simulink model "muscleLegs_task1"  (R2025b)
settings: Solver=ode23t  StartTime=0.0  StopTime=t_end  MaxStep=1e-3  RelTol=1e-4
values from neighbouring files (symbols this model uses):
  c = 0.05    [setup_muscleLegs_nm.m]
  CtrlPar = [tau_H_st; phi_K_tgt_st; P_K_st; D_K_st ... (first row only)    [setup_muscleLegs_ctrl.m]
  eref_se = 0.04    [setup_muscleLegs_nm.m]
  FmaxBFSH = 350    [setup_muscleLegs_nm.m]
  FmaxGLU = 4000    [setup_muscleLegs_nm.m]
  FmaxHFL = 2000    [setup_muscleLegs_nm.m]
  FmaxVAS = 5000    [setup_muscleLegs_nm.m]
  g = 9.81    [setup_muscleLegs_model.m]
  init_stim = 0.01    [setup_muscleLegs_nm.m]
  K = 5    [setup_muscleLegs_nm.m]
  l_shank = l_leg/2    (= 0.49)    [setup_muscleLegs_model.m]
  l_thigh = l_leg/2    (= 0.49)    [setup_muscleLegs_model.m]
  loptBFSH = 0.12    [setup_muscleLegs_nm.m]
  loptGLU = 0.11    [setup_muscleLegs_nm.m]
  loptHFL = 0.11    [setup_muscleLegs_nm.m]
  loptVAS = 0.08    [setup_muscleLegs_nm.m]
  lslackBFSH = 0.10    (= 0.1)    [setup_muscleLegs_nm.m]
  lslackGLU = 0.13    [setup_muscleLegs_nm.m]
  lslackHFL = 0.10    (= 0.1)    [setup_muscleLegs_nm.m]
  lslackVAS = 0.23    [setup_muscleLegs_nm.m]
  m_body = m_total - 2*m_foot    (= 78)    [setup_muscleLegs_model.m]
  m_shank = 4    [setup_muscleLegs_model.m]
  m_thigh = 8    [setup_muscleLegs_model.m]
  N = 12    [cmaes_task1_2_set1.mat]    (also in cmaes_task1_2_set2.mat; cmaes_task2_2_set1.mat = 17; cmaes_task2_2_set2.mat = 17; cmaes_task3_crouch.mat = 17)
  phirefBFSH = 160*pi/180    (= 2.79252680319)    [setup_muscleLegs_nm.m]
  phirefGLU = 60*pi/180    (= 1.0471975512)    [setup_muscleLegs_nm.m]
  phirefHFL = 20*pi/180    (= 0.349065850399)    [setup_muscleLegs_nm.m]
  phirefVAS = 60*pi/180    (= 1.0471975512)    [setup_muscleLegs_nm.m]
  plane_height = 0.1    [setup_muscleLegs_model.m]
  plane_x = 100    [setup_muscleLegs_model.m]
  plane_z = 1    [setup_muscleLegs_model.m]
  r_foot = 0.01    [setup_muscleLegs_model.m]
  rBFSH = 0.04    [setup_muscleLegs_nm.m]
  rGLU = 0.08    [setup_muscleLegs_nm.m]
  rHFL = 0.08    [setup_muscleLegs_nm.m]
  rhoBFSH = 0.7    [setup_muscleLegs_nm.m]
  rhoGLU = 0.5    [setup_muscleLegs_nm.m]
  rhoHFL = 0.5    [setup_muscleLegs_nm.m]
  rhoVAS = 0.6    [setup_muscleLegs_nm.m]
  rVAS = 0.05    [setup_muscleLegs_nm.m]
  tau_act = 0.01    [setup_muscleLegs_nm.m]
  tau_deact = 0.04    [setup_muscleLegs_nm.m]
  vi_Ctrl_st = 1:4    [setup_muscleLegs_ctrl.m]
  vi_Ctrl_sw = 5:12    [setup_muscleLegs_ctrl.m]
  vmaxBFSH = 12    [setup_muscleLegs_nm.m]
  vmaxGLU = 12    [setup_muscleLegs_nm.m]
  vmaxHFL = 12    [setup_muscleLegs_nm.m]
  vmaxVAS = 12    [setup_muscleLegs_nm.m]
  w = 0.56    [setup_muscleLegs_nm.m]
  w_pe = w    (= 0.56)    [setup_muscleLegs_nm.m]
undefined symbols (not defined in the file or in its folder): l1, X, Y, Z
libraries: sm_lib x30, nesl_utility x17, simulink x1
(part 1 of 4)
settings Model: Creator=ssm04  LastModifiedBy=mayan
settings SolverCC: AlgebraicLoopSolver=TrustRegion
settings OptimizationCC: ReuseModelBlockBuffer=off
settings RTWCC: GPUComputeCapability=3.5
settings ExplorerConfigSet: InternalSimMechanicsExplorerSettings="<ExplorerConfiguration><canonicalview>planar_xy</canonicalview><AnimationSetting><BasePlaybackSpeed>1.0</BasePlaybackSpeed><PlaybackSpeedFactor>1.0</PlaybackSpeedFactor></AnimationSetting><TilePanel><TileInfo><Tiles Columns=\"1\" Count=\"1\" Rows=\"1\"><Column Weight=\"1\"/><Row Weight=\"1\"/><Tile Height=\"1\" Width=\"1\" X=\"0\" Y=\"0\"/></Tiles></TileInfo><SceneInfo><SceneViewer><BGColor><R>0.60000002384185791</R><G>0.60000002384185791</G><B>0.60000002384185791</B></BGColor><Camera><DoPerspective>off</DoPerspective><Position><X>5.32836294698793811</X><Y>0.88627330653474079</Y><Z>5.31412817539694871</Z></Position><Center><X>5.32836294698793811</X><Y>0.88627330653474079</Y><Z>2.38238317962213841e-09</Z></Center><Up><X>0</X><Y>1</Y><Z>0</Z></Up><ViewLimDist>1</ViewLimDist><YLim>2.08582257526475079</YLim><XLim>5.52596682264529182</XLim></Camera></SceneViewer></SceneInfo></TilePanel><MechEditorPanel><Cameras/><GfxPanelCameraMap/><VideoCreator><PlaybackSpeedRatio>1.0</PlaybackSpeedRatio><FrameRate>30</FrameRate><VideoFormat>Motion JPEG AVI</VideoFormat><FrameSize>auto</FrameSize></VideoCreator></MechEditorPanel></ExplorerConfiguration>"

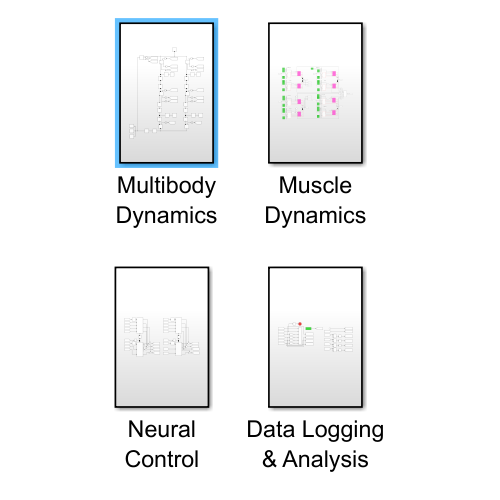
[thumbnail: Simulink's stored preview of the top-level diagram]
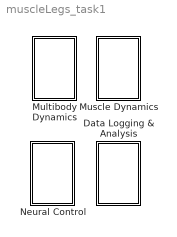
== system muscleLegs_task1 ==
  Data Logging & Analysis : Subsystem
  Multibody Dynamics : Subsystem
  Muscle Dynamics : Subsystem
  Neural Control : Subsystem

== system muscleLegs_task1/Data Logging & Analysis ==
  Clock : Clock
  Compare To Constant : simulink/Logic and Bit Operations/Compare To Constant  relop=<=  const=0.5  OutDataTypeStr=boolean
  Constant3 : Constant  Value=CtrlPar
  Divide{1..4} (4 alike) : Product
  Gain{,1..3} (4 alike) : Gain  Gain=180/pi
  Integrator{,1..3} (4 alike) : Integrator
  Scope1 : Scope  NumInputPorts=6
      settings: ActiveDisplayYMinimum=0.94241  ActiveDisplayYMaximum=1.51828
  Stop Simulation : Stop
  To Workspace : ToWorkspace  VariableName=t_end_sim  SaveFormat=Timeseries  SampleTime=-1
      settings: MaxDataPoints=1
  To Workspace1 : ToWorkspace  VariableName=x_end  SaveFormat=Timeseries  SampleTime=-1
      settings: MaxDataPoints=1
  To Workspace2 : ToWorkspace  VariableName=int_tau_H_L_2  SaveFormat=Timeseries  SampleTime=-1
      settings: MaxDataPoints=1
  To Workspace3 : ToWorkspace  VariableName=int_tau_K_L_2  SaveFormat=Timeseries  SampleTime=-1
      settings: MaxDataPoints=1
  To Workspace4 : ToWorkspace  VariableName=int_tau_H_R_2  SaveFormat=Timeseries  SampleTime=-1
      settings: MaxDataPoints=1
  To Workspace5 : ToWorkspace  VariableName=int_tau_K_R_2  SaveFormat=Timeseries  SampleTime=-1
      settings: MaxDataPoints=1
  To Workspace6 : ToWorkspace  VariableName=log_phi_H_L  SaveFormat=Timeseries  SampleTime=-1
  To Workspace7 : ToWorkspace  VariableName=log_phi_H_R  SaveFormat=Timeseries  SampleTime=-1
  To Workspace8 : ToWorkspace  VariableName=log_phi_K_L  SaveFormat=Timeseries  SampleTime=-1
  To Workspace9 : ToWorkspace  VariableName=log_phi_K_R  SaveFormat=Timeseries  SampleTime=-1
  tag scope: CtrlPar=global
  wires:
  Gain3/1 -> Scope1/6  "k_R"
  [body_y] -> Compare To Constant/1, Scope1/2
  [phi_K_L] -> To Workspace8/1, Gain1/1
  [tau_K_R] -> Divide3/2, Divide3/1
  Compare To Constant/1 -> Stop Simulation/1
  [phi_H_L] -> To Workspace6/1, Gain/1
  Integrator1/1 -> To Workspace3/1
  [phi_K_R] -> To Workspace9/1, Gain3/1
  [body_x] -> Scope1/1
  [tau_H_L] -> Divide2/2, Divide2/1
  Gain2/1 -> Scope1/5  "h_R"
  Gain/1 -> Scope1/3  "h_L"
  [phi_H_R] -> To Workspace7/1, Gain2/1
  [body_x] -> To Workspace1/1
  Clock/1 -> To Workspace/1
  Constant3/1 -> [CtrlPar]
  [tau_K_L] -> Divide1/2, Divide1/1
  Divide2/1 -> Integrator/1
  [tau_H_R] -> Divide4/2, Divide4/1
  Divide1/1 -> Integrator1/1
  Integrator3/1 -> To Workspace5/1
  Integrator2/1 -> To Workspace4/1
  Gain1/1 -> Scope1/4  "k_L"
  Divide4/1 -> Integrator2/1
  Integrator/1 -> To Workspace2/1
  Divide3/1 -> Integrator3/1

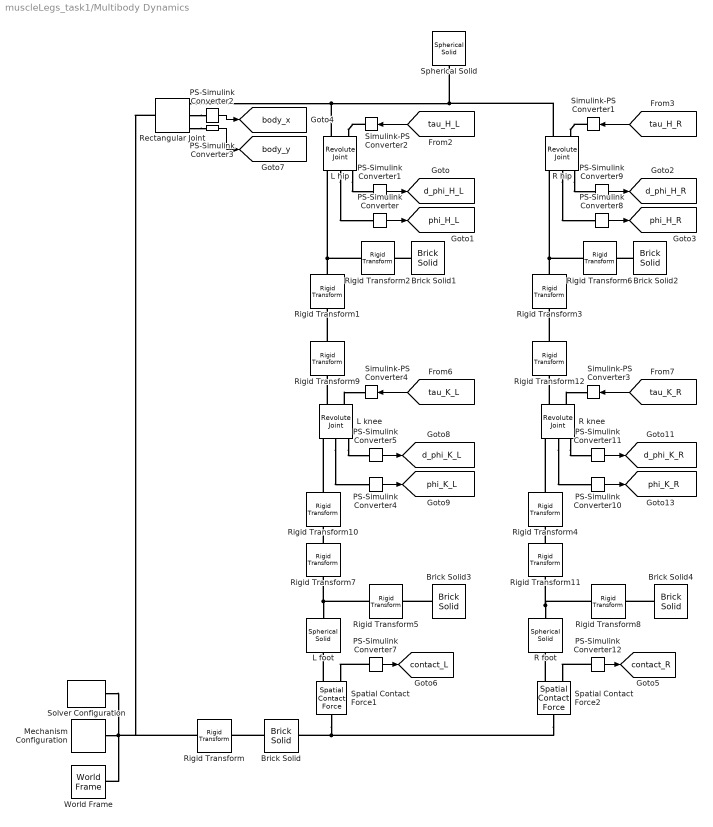
== system muscleLegs_task1/Multibody Dynamics ==
  Brick Solid : sm_lib/Body Elements/Brick Solid  BrickDimensions=[plane_x plane_height plane_z]  BrickDimensionsUnits=m  ExportEntireGeometry=on  InertiaType=CalculateFromGeometry  BasedOnType=Density  Density=1000  DensityUnits=kg/m^3  Mass=1  MassUnits=kg  CenterOfMass=[0 0 0]  CenterOfMassUnits=m  MomentsOfInertia=[1 1 1]  MomentsOfInertiaUnits=kg*m^2  ProductsOfInertia=[0 0 0]  ProductsOfInertiaUnits=kg*m^2  GraphicType=FromGeometry  MarkerShape=Sphere  MarkerSize=10  GraphicVisPropType=SimpleVisualProperties  GraphicDiffuseColor=[0.5 0.5 0.5]  GraphicOpacity=1.0  GraphicSpecularColor=[0.5 0.5 0.5 1.0]  GraphicAmbientColor=[0.15 0.15 0.15 1.0]  GraphicEmissiveColor=[0.0 0.0 0.0 1.0]  GraphicShininess=75  DoExposeReferenceFrame=on  SerializedFrames=<Frames/>
  Brick Solid1 : sm_lib/Body Elements/Brick Solid  BrickDimensions=[0.08 l_thigh 0.08]  BrickDimensionsUnits=m  ExportEntireGeometry=off  InertiaType=Custom  BasedOnType=Density  Density=0  DensityUnits=kg/m^3  Mass=m_thigh  MassUnits=kg  CenterOfMass=com_thigh  CenterOfMassUnits=m  MomentsOfInertia=I_thigh  MomentsOfInertiaUnits=kg*m^2  ProductsOfInertia=[0 0 0]  ProductsOfInertiaUnits=kg*m^2  GraphicType=FromGeometry  MarkerShape=Sphere  MarkerSize=10  GraphicVisPropType=SimpleVisualProperties  GraphicDiffuseColor=[0.6 0.0 0.0]  GraphicOpacity=1  GraphicSpecularColor=[0.5 0.5 0.5 1.0]  GraphicAmbientColor=[0.15 0.15 0.15 1.0]  GraphicEmissiveColor=[0.0 0.0 0.0 1.0]  GraphicShininess=75  DoExposeReferenceFrame=on  SerializedFrames=<Frames/>
  Brick Solid2 : sm_lib/Body Elements/Brick Solid  BrickDimensions=[0.08 l_thigh 0.08]  BrickDimensionsUnits=m  ExportEntireGeometry=off  InertiaType=Custom  BasedOnType=Density  Density=0  DensityUnits=kg/m^3  Mass=m_thigh  MassUnits=kg  CenterOfMass=com_thigh  CenterOfMassUnits=m  MomentsOfInertia=I_thigh  MomentsOfInertiaUnits=kg*m^2  ProductsOfInertia=[0 0 0]  ProductsOfInertiaUnits=kg*m^2  GraphicType=FromGeometry  MarkerShape=Sphere  MarkerSize=10  GraphicVisPropType=SimpleVisualProperties  GraphicDiffuseColor=[0.0 0.0 0.6]  GraphicOpacity=1  GraphicSpecularColor=[0.5 0.5 0.5 1.0]  GraphicAmbientColor=[0.15 0.15 0.15 1.0]  GraphicEmissiveColor=[0.0 0.0 0.0 1.0]  GraphicShininess=75  DoExposeReferenceFrame=on  SerializedFrames=<Frames/>
  Brick Solid3 : sm_lib/Body Elements/Brick Solid  BrickDimensions=[0.04 l_shank+r_foot 0.04]  BrickDimensionsUnits=m  ExportEntireGeometry=off  InertiaType=Custom  BasedOnType=Density  Density=0  DensityUnits=kg/m^3  Mass=m_shank  MassUnits=kg  CenterOfMass=com_shank  CenterOfMassUnits=m  MomentsOfInertia=I_shank  MomentsOfInertiaUnits=kg*m^2  ProductsOfInertia=[0 0 0]  ProductsOfInertiaUnits=kg*m^2  GraphicType=FromGeometry  MarkerShape=Sphere  MarkerSize=10  GraphicVisPropType=SimpleVisualProperties  GraphicDiffuseColor=[0.6 0.0 0.0]  GraphicOpacity=1  GraphicSpecularColor=[0.5 0.5 0.5 1.0]  GraphicAmbientColor=[0.15 0.15 0.15 1.0]  GraphicEmissiveColor=[0.0 0.0 0.0 1.0]  GraphicShininess=75  DoExposeReferenceFrame=on  SerializedFrames=<Frames/>
  Brick Solid4 : sm_lib/Body Elements/Brick Solid  BrickDimensions=[0.04 l_shank+r_foot 0.04]  BrickDimensionsUnits=m  ExportEntireGeometry=off  InertiaType=Custom  BasedOnType=Density  Density=0  DensityUnits=kg/m^3  Mass=1  MassUnits=kg  CenterOfMass=com_shank  CenterOfMassUnits=m  MomentsOfInertia=I_shank  MomentsOfInertiaUnits=kg*m^2  ProductsOfInertia=[0 0 0]  ProductsOfInertiaUnits=kg*m^2  GraphicType=FromGeometry  MarkerShape=Sphere  MarkerSize=10  GraphicVisPropType=SimpleVisualProperties  GraphicDiffuseColor=[0.0 0.0 0.6]  GraphicOpacity=1  GraphicSpecularColor=[0.5 0.5 0.5 1.0]  GraphicAmbientColor=[0.15 0.15 0.15 1.0]  GraphicEmissiveColor=[0.0 0.0 0.0 1.0]  GraphicShininess=75  DoExposeReferenceFrame=on  SerializedFrames=<Frames/>
  L foot : sm_lib/Body Elements/Spherical Solid  SphereRadius=r_foot  SphereRadiusUnits=m  ExportEntireGeometry=on  InertiaType=PointMass  BasedOnType=Density  Density=1000  DensityUnits=kg/m^3  Mass=1  MassUnits=kg  CenterOfMass=[0 0 0]  CenterOfMassUnits=m  MomentsOfInertia=[1 1 1]  MomentsOfInertiaUnits=kg*m^2  ProductsOfInertia=[0 0 0]  ProductsOfInertiaUnits=kg*m^2  GraphicType=FromGeometry  MarkerShape=Sphere  MarkerSize=10  GraphicVisPropType=SimpleVisualProperties  GraphicDiffuseColor=[0.5 0.5 0.5]  GraphicOpacity=1.0  GraphicSpecularColor=[0.5 0.5 0.5 1.0]  GraphicAmbientColor=[0.15 0.15 0.15 1.0]  GraphicEmissiveColor=[0.0 0.0 0.0 1.0]  GraphicShininess=75  DoExposeReferenceFrame=on  SerializedFrames=<Frames/>
  L hip : sm_lib/Joints/Revolute Joint  JointMode=Normal  CompositeWrenchDir=FollowerOnBase  CompositeWrenchFrame=BaseFrame  SenseConstraintForce=off  SenseConstraintTorque=off  SenseTotalForce=off  SenseTotalTorque=off  PositionTargetSpecify=on  PositionTargetPriority=High  PositionTargetValue=phi0_H_L  PositionTargetValueUnits=rad  VelocityTargetSpecify=on  VelocityTargetPriority=High  VelocityTargetValue=d_phi0_H_L  VelocityTargetValueUnits=rad/s  EquilibriumPosition=0  EquilibriumPositionUnits=deg  SpringStiffness=0  SpringStiffnessUnits=N*m/deg  DampingCoefficient=0  DampingCoefficientUnits=N*m/(deg/s)  LowerLimitSpecify=off  LowerLimitBound=-90  LowerLimitBoundUnits=deg  LowerLimitStiffness=1e4  LowerLimitStiffnessUnits=N*m/deg  LowerLimitDamping=10  LowerLimitDampingUnits=N*m/(deg/s)  LowerLimitTransitionRegionWidth=0.1  LowerLimitTransitionRegionWidthUnits=deg  UpperLimitSpecify=off  UpperLimitBound=90  UpperLimitBoundUnits=deg  UpperLimitStiffness=1e4  UpperLimitStiffnessUnits=N*m/deg  UpperLimitDamping=10  UpperLimitDampingUnits=N*m/(deg/s)  UpperLimitTransitionRegionWidth=0.1  UpperLimitTransitionRegionWidthUnits=deg  TorqueActuationMode=InputTorque  MotionActuationMode=ComputedMotion  SensePosition=on  SenseVelocity=on  SenseAcceleration=off  SenseTorqueForce=off  SenseLowerLimitTorqueForce=off  SenseUpperLimitTorqueForce=off
  L knee : sm_lib/Joints/Revolute Joint  JointMode=Normal  CompositeWrenchDir=FollowerOnBase  CompositeWrenchFrame=BaseFrame  SenseConstraintForce=off  SenseConstraintTorque=off  SenseTotalForce=off  SenseTotalTorque=off  PositionTargetSpecify=on  PositionTargetPriority=High  PositionTargetValue=phi0_K_L  PositionTargetValueUnits=rad  VelocityTargetSpecify=off  VelocityTargetPriority=High  VelocityTargetValue=d_phi0_L  VelocityTargetValueUnits=rad/s  EquilibriumPosition=0  EquilibriumPositionUnits=deg  SpringStiffness=0  SpringStiffnessUnits=N*m/deg  DampingCoefficient=0  DampingCoefficientUnits=N*m/(deg/s)  LowerLimitSpecify=on  LowerLimitBound=del_phi_K  LowerLimitBoundUnits=rad  LowerLimitStiffness=1e4  LowerLimitStiffnessUnits=N*m/deg  LowerLimitDamping=10  LowerLimitDampingUnits=N*m/(deg/s)  LowerLimitTransitionRegionWidth=0.1  LowerLimitTransitionRegionWidthUnits=deg  UpperLimitSpecify=off  UpperLimitBound=90  UpperLimitBoundUnits=deg  UpperLimitStiffness=1e4  UpperLimitStiffnessUnits=N*m/deg  UpperLimitDamping=10  UpperLimitDampingUnits=N*m/(deg/s)  UpperLimitTransitionRegionWidth=0.1  UpperLimitTransitionRegionWidthUnits=deg  TorqueActuationMode=InputTorque  MotionActuationMode=ComputedMotion  SensePosition=on  SenseVelocity=on  SenseAcceleration=off  SenseTorqueForce=off  SenseLowerLimitTorqueForce=off  SenseUpperLimitTorqueForce=off
  Mechanism Configuration : sm_lib/Utilities/Mechanism Configuration  UniformGravity=Constant  GravityVector=[0 -g 0]  GravityVectorUnits=m/s^2  LinearizationDelta=0.001  JointModeTransitionNonlinearIterations=2
  PS-Simulink Converter{,1..5,7..12} (12 alike) : nesl_utility/PS-Simulink Converter  PhysicalDomain=network_engine_domain  SubClassName=ps_output  LeftPortType=input  RightPortType=output  PseudoPeriodic=off  Frequencies=[]  VectorFormat=inherit  Unit=inherit  AffineConversion=off
  R foot : sm_lib/Body Elements/Spherical Solid  SphereRadius=r_foot  SphereRadiusUnits=m  ExportEntireGeometry=on  InertiaType=PointMass  BasedOnType=Density  Density=1000  DensityUnits=kg/m^3  Mass=1  MassUnits=kg  CenterOfMass=[0 0 0]  CenterOfMassUnits=m  MomentsOfInertia=[1 1 1]  MomentsOfInertiaUnits=kg*m^2  ProductsOfInertia=[0 0 0]  ProductsOfInertiaUnits=kg*m^2  GraphicType=FromGeometry  MarkerShape=Sphere  MarkerSize=10  GraphicVisPropType=SimpleVisualProperties  GraphicDiffuseColor=[0.5 0.5 0.5]  GraphicOpacity=1.0  GraphicSpecularColor=[0.5 0.5 0.5 1.0]  GraphicAmbientColor=[0.15 0.15 0.15 1.0]  GraphicEmissiveColor=[0.0 0.0 0.0 1.0]  GraphicShininess=75  DoExposeReferenceFrame=on  SerializedFrames=<Frames/>
  R hip : sm_lib/Joints/Revolute Joint  JointMode=Normal  CompositeWrenchDir=FollowerOnBase  CompositeWrenchFrame=BaseFrame  SenseConstraintForce=off  SenseConstraintTorque=off  SenseTotalForce=off  SenseTotalTorque=off  PositionTargetSpecify=on  PositionTargetPriority=High  PositionTargetValue=phi0_H_R  PositionTargetValueUnits=rad  VelocityTargetSpecify=on  VelocityTargetPriority=High  VelocityTargetValue=d_phi0_H_R  VelocityTargetValueUnits=rad/s  EquilibriumPosition=0  EquilibriumPositionUnits=deg  SpringStiffness=0  SpringStiffnessUnits=N*m/deg  DampingCoefficient=0  DampingCoefficientUnits=N*m/(deg/s)  LowerLimitSpecify=off  LowerLimitBound=-90  LowerLimitBoundUnits=deg  LowerLimitStiffness=1e4  LowerLimitStiffnessUnits=N*m/deg  LowerLimitDamping=10  LowerLimitDampingUnits=N*m/(deg/s)  LowerLimitTransitionRegionWidth=0.1  LowerLimitTransitionRegionWidthUnits=deg  UpperLimitSpecify=off  UpperLimitBound=90  UpperLimitBoundUnits=deg  UpperLimitStiffness=1e4  UpperLimitStiffnessUnits=N*m/deg  UpperLimitDamping=10  UpperLimitDampingUnits=N*m/(deg/s)  UpperLimitTransitionRegionWidth=0.1  UpperLimitTransitionRegionWidthUnits=deg  TorqueActuationMode=InputTorque  MotionActuationMode=ComputedMotion  SensePosition=on  SenseVelocity=on  SenseAcceleration=off  SenseTorqueForce=off  SenseLowerLimitTorqueForce=off  SenseUpperLimitTorqueForce=off
  R knee : sm_lib/Joints/Revolute Joint  JointMode=Normal  CompositeWrenchDir=FollowerOnBase  CompositeWrenchFrame=BaseFrame  SenseConstraintForce=off  SenseConstraintTorque=off  SenseTotalForce=off  SenseTotalTorque=off  PositionTargetSpecify=on  PositionTargetPriority=High  PositionTargetValue=phi0_K_R  PositionTargetValueUnits=rad  VelocityTargetSpecify=off  VelocityTargetPriority=High  VelocityTargetValue=d_phi0_L  VelocityTargetValueUnits=rad/s  EquilibriumPosition=0  EquilibriumPositionUnits=deg  SpringStiffness=0  SpringStiffnessUnits=N*m/deg  DampingCoefficient=0  DampingCoefficientUnits=N*m/(deg/s)  LowerLimitSpecify=on  LowerLimitBound=del_phi_K  LowerLimitBoundUnits=rad  LowerLimitStiffness=1e4  LowerLimitStiffnessUnits=N*m/deg  LowerLimitDamping=10  LowerLimitDampingUnits=N*m/(deg/s)  LowerLimitTransitionRegionWidth=0.1  LowerLimitTransitionRegionWidthUnits=deg  UpperLimitSpecify=off  UpperLimitBound=90  UpperLimitBoundUnits=deg  UpperLimitStiffness=1e4  UpperLimitStiffnessUnits=N*m/deg  UpperLimitDamping=10  UpperLimitDampingUnits=N*m/(deg/s)  UpperLimitTransitionRegionWidth=0.1  UpperLimitTransitionRegionWidthUnits=deg  TorqueActuationMode=InputTorque  MotionActuationMode=ComputedMotion  SensePosition=on  SenseVelocity=on  SenseAcceleration=off  SenseTorqueForce=off  SenseLowerLimitTorqueForce=off  SenseUpperLimitTorqueForce=off
  Rectangular Joint : sm_lib/Joints/Rectangular Joint  JointMode=Normal  CompositeWrenchDir=FollowerOnBase  CompositeWrenchFrame=BaseFrame  SenseConstraintForce=off  SenseConstraintTorque=off  SenseTotalForce=off  SenseTotalTorque=off  PxPositionTargetSpecify=on  PxPositionTargetPriority=High  PxPositionTargetValue=x0  PxPositionTargetValueUnits=m  PxVelocityTargetSpecify=on  PxVelocityTargetPriority=High  PxVelocityTargetValue=d_x0  PxVelocityTargetValueUnits=m/s  PxEquilibriumPosition=0  PxEquilibriumPositionUnits=m  PxSpringStiffness=0  PxSpringStiffnessUnits=N/m  PxDampingCoefficient=0  PxDampingCoefficientUnits=N/(m/s)  PxLowerLimitSpecify=off  PxLowerLimitBound=-1  PxLowerLimitBoundUnits=m  PxLowerLimitStiffness=1e6  PxLowerLimitStiffnessUnits=N/m  PxLowerLimitDamping=1e3  PxLowerLimitDampingUnits=N/(m/s)  PxLowerLimitTransitionRegionWidth=1e-4  PxLowerLimitTransitionRegionWidthUnits=m  PxUpperLimitSpecify=off  PxUpperLimitBound=1  PxUpperLimitBoundUnits=m  PxUpperLimitStiffness=1e6  PxUpperLimitStiffnessUnits=N/m  PxUpperLimitDamping=1e3  PxUpperLimitDampingUnits=N/(m/s)  PxUpperLimitTransitionRegionWidth=1e-4  PxUpperLimitTransitionRegionWidthUnits=m  PxTorqueActuationMode=NoTorque  PxMotionActuationMode=ComputedMotion  PxSensePosition=on  PxSenseVelocity=off  PxSenseAcceleration=off  PxSenseTorqueForce=off  PxSenseLowerLimitTorqueForce=off  PxSenseUpperLimitTorqueForce=off  PyPositionTargetSpecify=on  PyPositionTargetPriority=High  PyPositionTargetValue=y0  PyPositionTargetValueUnits=m  PyVelocityTargetSpecify=on  PyVelocityTargetPriority=High  PyVelocityTargetValue=d_y0  PyVelocityTargetValueUnits=m/s  PyEquilibriumPosition=0  PyEquilibriumPositionUnits=m  PySpringStiffness=0  PySpringStiffnessUnits=N/m  PyDampingCoefficient=0  PyDampingCoefficientUnits=N/(m/s)  PyLowerLimitSpecify=off  PyLowerLimitBound=-1  PyLowerLimitBoundUnits=m  PyLowerLimitStiffness=1e6  PyLowerLimitStiffnessUnits=N/m  PyLowerLimitDamping=1e3  PyLowerLimitDampingUnits=N/(m/s)  PyLowerLimitTransitionRegionWidth=1e-4  PyLowerLimitTransitionRegionWidthUnits=m  PyUpperLimitSpecify=off  PyUpperLimitBound=1  PyUpperLimitBoundUnits=m  PyUpperLimitStiffness=1e6  PyUpperLimitStiffnessUnits=N/m  PyUpperLimitDamping=1e3  PyUpperLimitDampingUnits=N/(m/s)  PyUpperLimitTransitionRegionWidth=1e-4  PyUpperLimitTransitionRegionWidthUnits=m  PyTorqueActuationMode=NoTorque  PyMotionActuationMode=ComputedMotion  PySensePosition=on  PySenseVelocity=off  PySenseAcceleration=off  PySenseTorqueForce=off  PySenseLowerLimitTorqueForce=off  PySenseUpperLimitTorqueForce=off
  Rigid Transform : sm_lib/Frames and Transforms/Rigid Transform  RotationMethod=None  FollAlignAxisA=+X  BaseAlignAxisA=+Y  FollAlignAxisB=+Y  BaseAlignAxisB=+Z  RotationStandardAxis=+Z  RotationAngle=0.0  RotationAngleUnits=deg  RotationArbitraryAxis=[0 0 1]  RotationSequenceAxes=FollowerAxes  RotationSequence=XYX  RotationSequenceAngles=[0 0 0]  RotationSequenceAnglesUnits=deg  RotationMatrix=[1 0 0; 0 1 0; 0 0 1]  Quaternion=[1 0 0 0]  TranslationMethod=Cartesian  TranslationCartesianOffset=[plane_x/2 -plane_height/2 0]  TranslationCartesianOffsetUnits=m  TranslationStandardAxis=-Y  TranslationStandardOffset=plane_height/2  TranslationStandardOffsetUnits=m  TranslationROffset=0  TranslationROffsetUnits=m  TranslationThetaOffset=0  TranslationThetaOffsetUnits=deg  TranslationZOffset=0  TranslationZOffsetUnits=m
  Rigid Transform1 : sm_lib/Frames and Transforms/Rigid Transform  RotationMethod=None  FollAlignAxisA=+Z  BaseAlignAxisA=-Z  FollAlignAxisB=+X  BaseAlignAxisB=+X  RotationStandardAxis=+Z  RotationAngle=0  RotationAngleUnits=deg  RotationArbitraryAxis=[0 0 1]  RotationSequenceAxes=FollowerAxes  RotationSequence=XYX  RotationSequenceAngles=[0 0 0]  RotationSequenceAnglesUnits=deg  RotationMatrix=[1 0 0;0 1 0;0 0 1]  Quaternion=[1 0 0 0]  TranslationMethod=Cartesian  TranslationCartesianOffset=[0 -l_thigh 0]  TranslationCartesianOffsetUnits=m  TranslationStandardAxis=-Y  TranslationStandardOffset=l1/2  TranslationStandardOffsetUnits=m  TranslationROffset=0  TranslationROffsetUnits=m  TranslationThetaOffset=0  TranslationThetaOffsetUnits=deg  TranslationZOffset=0  TranslationZOffsetUnits=m
  Rigid Transform10 : sm_lib/Frames and Transforms/Rigid Transform  RotationMethod=AlignedAxes  FollAlignAxisA=+Z  BaseAlignAxisA=-Z  FollAlignAxisB=+X  BaseAlignAxisB=+X  RotationStandardAxis=+Z  RotationAngle=0  RotationAngleUnits=deg  RotationArbitraryAxis=[0 0 1]  RotationSequenceAxes=FollowerAxes  RotationSequence=XYX  RotationSequenceAngles=[0 0 0]  RotationSequenceAnglesUnits=deg  RotationMatrix=[1 0 0;0 1 0;0 0 1]  Quaternion=[1 0 0 0]  TranslationMethod=None  TranslationCartesianOffset=[0 -l_shank/2 0]  TranslationCartesianOffsetUnits=m  TranslationStandardAxis=-Y  TranslationStandardOffset=l1/2  TranslationStandardOffsetUnits=m  TranslationROffset=0  TranslationROffsetUnits=m  TranslationThetaOffset=0  TranslationThetaOffsetUnits=deg  TranslationZOffset=0  TranslationZOffsetUnits=m
  Rigid Transform11 : sm_lib/Frames and Transforms/Rigid Transform  RotationMethod=None  FollAlignAxisA=+Z  BaseAlignAxisA=-Z  FollAlignAxisB=+X  BaseAlignAxisB=+X  RotationStandardAxis=+Z  RotationAngle=0  RotationAngleUnits=deg  RotationArbitraryAxis=[0 0 1]  RotationSequenceAxes=FollowerAxes  RotationSequence=XYX  RotationSequenceAngles=[0 0 0]  RotationSequenceAnglesUnits=deg  RotationMatrix=[1 0 0;0 1 0;0 0 1]  Quaternion=[1 0 0 0]  TranslationMethod=Cartesian  TranslationCartesianOffset=[0 -l_shank-r_foot 0]  TranslationCartesianOffsetUnits=m  TranslationStandardAxis=-Y  TranslationStandardOffset=l1/2  TranslationStandardOffsetUnits=m  TranslationROffset=0  TranslationROffsetUnits=m  TranslationThetaOffset=0  TranslationThetaOffsetUnits=deg  TranslationZOffset=0  TranslationZOffsetUnits=m
  Rigid Transform12 : sm_lib/Frames and Transforms/Rigid Transform  RotationMethod=AlignedAxes  FollAlignAxisA=+Z  BaseAlignAxisA=-Z  FollAlignAxisB=+X  BaseAlignAxisB=+X  RotationStandardAxis=+Z  RotationAngle=0  RotationAngleUnits=deg  RotationArbitraryAxis=[0 0 1]  RotationSequenceAxes=FollowerAxes  RotationSequence=XYX  RotationSequenceAngles=[0 0 0]  RotationSequenceAnglesUnits=deg  RotationMatrix=[1 0 0;0 1 0;0 0 1]  Quaternion=[1 0 0 0]  TranslationMethod=None  TranslationCartesianOffset=[0 -l_thigh/2 0]  TranslationCartesianOffsetUnits=m  TranslationStandardAxis=-Y  TranslationStandardOffset=l1/2  TranslationStandardOffsetUnits=m  TranslationROffset=0  TranslationROffsetUnits=m  TranslationThetaOffset=0  TranslationThetaOffsetUnits=deg  TranslationZOffset=0  TranslationZOffsetUnits=m
  Rigid Transform2 : sm_lib/Frames and Transforms/Rigid Transform  RotationMethod=None  FollAlignAxisA=+X  BaseAlignAxisA=+Y  FollAlignAxisB=+Y  BaseAlignAxisB=+Z  RotationStandardAxis=+Z  RotationAngle=0  RotationAngleUnits=deg  RotationArbitraryAxis=[0 0 1]  RotationSequenceAxes=FollowerAxes  RotationSequence=XYX  RotationSequenceAngles=[0 0 0]  RotationSequenceAnglesUnits=deg  RotationMatrix=[1 0 0;0 1 0;0 0 1]  Quaternion=[1 0 0 0]  TranslationMethod=Cartesian  TranslationCartesianOffset=[0 -l_thigh/2 0]  TranslationCartesianOffsetUnits=m  TranslationStandardAxis=-Y  TranslationStandardOffset=l1/2  TranslationStandardOffsetUnits=m  TranslationROffset=0  TranslationROffsetUnits=m  TranslationThetaOffset=0  TranslationThetaOffsetUnits=deg  TranslationZOffset=0  TranslationZOffsetUnits=m
  Rigid Transform3 : sm_lib/Frames and Transforms/Rigid Transform  RotationMethod=None  FollAlignAxisA=+Z  BaseAlignAxisA=-Z  FollAlignAxisB=+X  BaseAlignAxisB=+X  RotationStandardAxis=+Z  RotationAngle=0  RotationAngleUnits=deg  RotationArbitraryAxis=[0 0 1]  RotationSequenceAxes=FollowerAxes  RotationSequence=XYX  RotationSequenceAngles=[0 0 0]  RotationSequenceAnglesUnits=deg  RotationMatrix=[1 0 0;0 1 0;0 0 1]  Quaternion=[1 0 0 0]  TranslationMethod=Cartesian  TranslationCartesianOffset=[0 -l_thigh 0]  TranslationCartesianOffsetUnits=m  TranslationStandardAxis=-Y  TranslationStandardOffset=l1/2  TranslationStandardOffsetUnits=m  TranslationROffset=0  TranslationROffsetUnits=m  TranslationThetaOffset=0  TranslationThetaOffsetUnits=deg  TranslationZOffset=0  TranslationZOffsetUnits=m
  Rigid Transform4 : sm_lib/Frames and Transforms/Rigid Transform  RotationMethod=AlignedAxes  FollAlignAxisA=+Z  BaseAlignAxisA=-Z  FollAlignAxisB=+X  BaseAlignAxisB=+X  RotationStandardAxis=+Z  RotationAngle=0  RotationAngleUnits=deg  RotationArbitraryAxis=[0 0 1]  RotationSequenceAxes=FollowerAxes  RotationSequence=XYX  RotationSequenceAngles=[0 0 0]  RotationSequenceAnglesUnits=deg  RotationMatrix=[1 0 0;0 1 0;0 0 1]  Quaternion=[1 0 0 0]  TranslationMethod=None  TranslationCartesianOffset=[0 -l_shank/2 0]  TranslationCartesianOffsetUnits=m  TranslationStandardAxis=-Y  TranslationStandardOffset=l1/2  TranslationStandardOffsetUnits=m  TranslationROffset=0  TranslationROffsetUnits=m  TranslationThetaOffset=0  TranslationThetaOffsetUnits=deg  TranslationZOffset=0  TranslationZOffsetUnits=m
  Rigid Transform5 : sm_lib/Frames and Transforms/Rigid Transform  RotationMethod=None  FollAlignAxisA=+Y  BaseAlignAxisA=+Z  FollAlignAxisB=+X  BaseAlignAxisB=+X  RotationStandardAxis=+Z  RotationAngle=0  RotationAngleUnits=deg  RotationArbitraryAxis=[0 0 1]  RotationSequenceAxes=FollowerAxes  RotationSequence=XYX  RotationSequenceAngles=[0 0 0]  RotationSequenceAnglesUnits=deg  RotationMatrix=[1 0 0;0 1 0;0 0 1]  Quaternion=[1 0 0 0]  TranslationMethod=Cartesian  TranslationCartesianOffset=[0 (l_shank+r_foot)/2 0]  TranslationCartesianOffsetUnits=m  TranslationStandardAxis=-Y  TranslationStandardOffset=l1/2  TranslationStandardOffsetUnits=m  TranslationROffset=0  TranslationROffsetUnits=m  TranslationThetaOffset=0  TranslationThetaOffsetUnits=deg  TranslationZOffset=0  TranslationZOffsetUnits=m
  Rigid Transform6 : sm_lib/Frames and Transforms/Rigid Transform  RotationMethod=None  FollAlignAxisA=+X  BaseAlignAxisA=+Y  FollAlignAxisB=+Y  BaseAlignAxisB=+Z  RotationStandardAxis=+Z  RotationAngle=0  RotationAngleUnits=deg  RotationArbitraryAxis=[0 0 1]  RotationSequenceAxes=FollowerAxes  RotationSequence=XYX  RotationSequenceAngles=[0 0 0]  RotationSequenceAnglesUnits=deg  RotationMatrix=[1 0 0;0 1 0;0 0 1]  Quaternion=[1 0 0 0]  TranslationMethod=Cartesian  TranslationCartesianOffset=[0 -l_thigh/2 0]  TranslationCartesianOffsetUnits=m  TranslationStandardAxis=-Y  TranslationStandardOffset=l1/2  TranslationStandardOffsetUnits=m  TranslationROffset=0  TranslationROffsetUnits=m  TranslationThetaOffset=0  TranslationThetaOffsetUnits=deg  TranslationZOffset=0  TranslationZOffsetUnits=m
  Rigid Transform7 : sm_lib/Frames and Transforms/Rigid Transform  RotationMethod=None  FollAlignAxisA=+Z  BaseAlignAxisA=-Z  FollAlignAxisB=+X  BaseAlignAxisB=+X  RotationStandardAxis=+Z  RotationAngle=0  RotationAngleUnits=deg  RotationArbitraryAxis=[0 0 1]  RotationSequenceAxes=FollowerAxes  RotationSequence=XYX  RotationSequenceAngles=[0 0 0]  RotationSequenceAnglesUnits=deg  RotationMatrix=[1 0 0;0 1 0;0 0 1]  Quaternion=[1 0 0 0]  TranslationMethod=Cartesian  TranslationCartesianOffset=[0 -l_shank-r_foot 0]  TranslationCartesianOffsetUnits=m  TranslationStandardAxis=-Y  TranslationStandardOffset=l1/2  TranslationStandardOffsetUnits=m  TranslationROffset=0  TranslationROffsetUnits=m  TranslationThetaOffset=0  TranslationThetaOffsetUnits=deg  TranslationZOffset=0  TranslationZOffsetUnits=m
  Rigid Transform8 : sm_lib/Frames and Transforms/Rigid Transform  RotationMethod=None  FollAlignAxisA=+Y  BaseAlignAxisA=+Z  FollAlignAxisB=+X  BaseAlignAxisB=+X  RotationStandardAxis=+Z  RotationAngle=0  RotationAngleUnits=deg  RotationArbitraryAxis=[0 0 1]  RotationSequenceAxes=FollowerAxes  RotationSequence=XYX  RotationSequenceAngles=[0 0 0]  RotationSequenceAnglesUnits=deg  RotationMatrix=[1 0 0;0 1 0;0 0 1]  Quaternion=[1 0 0 0]  TranslationMethod=Cartesian  TranslationCartesianOffset=[0 (l_shank+r_foot)/2 0]  TranslationCartesianOffsetUnits=m  TranslationStandardAxis=-Y  TranslationStandardOffset=l1/2  TranslationStandardOffsetUnits=m  TranslationROffset=0  TranslationROffsetUnits=m  TranslationThetaOffset=0  TranslationThetaOffsetUnits=deg  TranslationZOffset=0  TranslationZOffsetUnits=m
  Rigid Transform9 : sm_lib/Frames and Transforms/Rigid Transform  RotationMethod=AlignedAxes  FollAlignAxisA=+Z  BaseAlignAxisA=-Z  FollAlignAxisB=+X  BaseAlignAxisB=+X  RotationStandardAxis=+Z  RotationAngle=0  RotationAngleUnits=deg  RotationArbitraryAxis=[0 0 1]  RotationSequenceAxes=FollowerAxes  RotationSequence=XYX  RotationSequenceAngles=[0 0 0]  RotationSequenceAnglesUnits=deg  RotationMatrix=[1 0 0;0 1 0;0 0 1]  Quaternion=[1 0 0 0]  TranslationMethod=None  TranslationCartesianOffset=[0 -l_thigh/2 0]  TranslationCartesianOffsetUnits=m  TranslationStandardAxis=-Y  TranslationStandardOffset=l1/2  TranslationStandardOffsetUnits=m  TranslationROffset=0  TranslationROffsetUnits=m  TranslationThetaOffset=0  TranslationThetaOffsetUnits=deg  TranslationZOffset=0  TranslationZOffsetUnits=m
  Simulink-PS Converter{1..4} (4 alike) : nesl_utility/Simulink-PS Converter  PhysicalDomain=network_engine_domain  SubClassName=ps_input  LeftPortType=input  RightPortType=output  PseudoPeriodic=off  Frequencies=[]  NoiseDistribution=none  NoiseParameters=[]  Unit=1  AffineConversion=off  FilteringAndDerivatives=provide  SimscapeFilterOrder=1  InputFilterTimeConstant=0.001  UdotUserProvided=0
  Solver Configuration : nesl_utility/Solver Configuration  PhysicalDomain=network_engine_domain  SubClassName=solver  LeftPortType=input  RightPortType=generic  Tones=[]  Harmonics=[]  SimulateNoise=off  Profile=off  UseLocalSampling=off  EnableSwitchedLinearOptims=on  FrequencyDomain=off  UseCCode=off  RelTol=0.001  AbsTol=0.001  MinStep=1e-09  ToWorkspace=off  RevertToSquareIcSolve=off  NumHomotopyIterations=100  PhasorMode=off  PhasorModeNumHarmonics=1  ConsistencySolver=NEWTON_XTOL_AFTER_FTOL  IndexReductionMethod=DerivativeReplacement  DoDC=off  ResidualTolerance=1e-09  ConsistencyTolSource=GLOBAL  ConsistencyAbsTol=0.001  ConsistencyRelTol=0.001  ConsistencyTolFactor=1e-9  UseLocalSolver=off  LocalSolverChoice=NE_BACKWARD_EULER_ADVANCER  ResolveIndetEquations=on  FunctionEvalNumThread=1  LocalSolverSampleTime=0.001  DoFixedCost=off  MaxNonlinIter=3  MaxModeIter=2  ComputeImpulses=off  ImpulseIterations=2  LinearAlgebra=auto  LinearAlgebraNumThread=0  EquationFormulation=NE_TIME_EF  DelaysMemoryBudget=1024  AutomaticFiltering=on  FilteringTimeConstant=0.001  PartitionStorageMethod=AS_NEEDED  PartitionMemoryBudget=1024  PartitionMethod=ROBUST  MultibodyUseLocalSolver=off  MultibodyLocalSolverChoice=ODE1  MultibodyLocalSolverSampleTime=0.001
  Spatial Contact Force1 : sm_lib/Forces and Torques/Spatial Contact Force  SenseSeparationDistance=off  NormalForceType=SmoothSpringDamper  NormalStiffness=1e6  NormalStiffnessUnits=N/m  NormalDamping=1e5  NormalDampingUnits=N/(m/s)  NormalTransitionRegionWidth=1e-4  NormalTransitionRegionWidthUnits=m  FrictionType=SmoothStickSlip  CoefficientOfStaticFriction=0.5  CoefficientOfDynamicFriction=0.3  FrictionalCriticalVelocity=1e-3  FrictionalCriticalVelocityUnits=m/s  SenseContactSignal=on  SensePenetrationDepth=off  SenseNormalVelocity=off  SenseTangentialVelocity=off  SensingForceTorqueDirection=BaseOnFollower  SensingForceTorqueResolutionFrame=ContactFrame  SenseNormalForce=off  SenseNormalForceMagnitude=off  SenseNormalTorque=off  SenseFrictionalForce=off  SenseFrictionalForceMagnitude=off  SenseFrictionalTorque=off  SenseTotalForce=off  SenseTotalTorque=off  SenseContactBaseRotation=off  SenseContactBaseTranslation=off  SenseContactFollowerRotation=off  SenseContactFollowerTranslation=off  ZeroCrossDetectContactStartAndEnd=off
  Spatial Contact Force2 : sm_lib/Forces and Torques/Spatial Contact Force  SenseSeparationDistance=off  NormalForceType=SmoothSpringDamper  NormalStiffness=1e6  NormalStiffnessUnits=N/m  NormalDamping=1e5  NormalDampingUnits=N/(m/s)  NormalTransitionRegionWidth=1e-4  NormalTransitionRegionWidthUnits=m  FrictionType=SmoothStickSlip  CoefficientOfStaticFriction=0.5  CoefficientOfDynamicFriction=0.3  FrictionalCriticalVelocity=1e-3  FrictionalCriticalVelocityUnits=m/s  SenseContactSignal=on  SensePenetrationDepth=off  SenseNormalVelocity=off  SenseTangentialVelocity=off  SensingForceTorqueDirection=BaseOnFollower  SensingForceTorqueResolutionFrame=ContactFrame  SenseNormalForce=off  SenseNormalForceMagnitude=off  SenseNormalTorque=off  SenseFrictionalForce=off  SenseFrictionalForceMagnitude=off  SenseFrictionalTorque=off  SenseTotalForce=off  SenseTotalTorque=off  SenseContactBaseRotation=off  SenseContactBaseTranslation=off  SenseContactFollowerRotation=off  SenseContactFollowerTranslation=off  ZeroCrossDetectContactStartAndEnd=off
  Spherical Solid : sm_lib/Body Elements/Spherical Solid  SphereRadius=0.1  SphereRadiusUnits=m  ExportEntireGeometry=off  InertiaType=PointMass  BasedOnType=Density  Density=1000  DensityUnits=kg/m^3  Mass=m_body  MassUnits=kg  CenterOfMass=[0 0 0]  CenterOfMassUnits=m  MomentsOfInertia=[1 1 1]  MomentsOfInertiaUnits=kg*m^2  ProductsOfInertia=[0 0 0]  ProductsOfInertiaUnits=kg*m^2  GraphicType=FromGeometry  MarkerShape=Sphere  MarkerSize=10  GraphicVisPropType=SimpleVisualProperties  GraphicDiffuseColor=[0.5 0.5 0.5]  GraphicOpacity=1.0  GraphicSpecularColor=[0.5 0.5 0.5 1.0]  GraphicAmbientColor=[0.15 0.15 0.15 1.0]  GraphicEmissiveColor=[0.0 0.0 0.0 1.0]  GraphicShininess=75  DoExposeReferenceFrame=on  SerializedFrames=<Frames/>
  World Frame : sm_lib/Frames and Transforms/World Frame
  tag scope: body_x=global, body_y=global, contact_L=global, contact_R=global, d_phi_H_L=global, d_phi_H_R=global, d_phi_K_L=global, d_phi_K_R=global, phi_H_L=global, phi_H_R=global, phi_K_L=global, phi_K_R=global
  wires:
  PS-Simulink Converter10/1 -> [phi_K_R]
  PS-Simulink Converter/1 -> [phi_H_L]
  PS-Simulink Converter8/1 -> [phi_H_R]
  PS-Simulink Converter12/1 -> [contact_R]
  [tau_H_L] -> Simulink-PS Converter2/1
  PS-Simulink Converter1/1 -> [d_phi_H_L]
  [tau_H_R] -> Simulink-PS Converter1/1
  PS-Simulink Converter7/1 -> [contact_L]
  [tau_K_L] -> Simulink-PS Converter4/1
  [tau_K_R] -> Simulink-PS Converter3/1
  PS-Simulink Converter5/1 -> [d_phi_K_L]
  PS-Simulink Converter2/1 -> [body_x]
  PS-Simulink Converter9/1 -> [d_phi_H_R]
  PS-Simulink Converter3/1 -> [body_y]
  PS-Simulink Converter11/1 -> [d_phi_K_R]
  PS-Simulink Converter4/1 -> [phi_K_L]
  connections:
  Solver Configuration/RConn1 -- Rectangular Joint/LConn1 -- Rigid Transform/LConn1 -- Mechanism Configuration/RConn1 -- World Frame/RConn1
  Brick Solid4/RConn1 -- Rigid Transform8/RConn1
  Brick Solid/RConn1 -- Rigid Transform/RConn1
  Brick Solid1/RConn1 -- Rigid Transform2/RConn1
  Spatial Contact Force1/LConn1 -- Spatial Contact Force2/LConn1 -- Brick Solid/LConn1
  Rectangular Joint/RConn1 -- L hip/LConn1 -- R hip/LConn1 -- Spherical Solid/RConn1
  Simulink-PS Converter2/RConn1 -- L hip/LConn2
  Brick Solid2/RConn1 -- Rigid Transform6/RConn1
  Rigid Transform6/LConn1 -- Rigid Transform3/LConn1 -- R hip/RConn1
  Rigid Transform12/LConn1 -- Rigid Transform3/RConn1
  L knee/RConn3 -- PS-Simulink Converter5/LConn1
  Spatial Contact Force1/RConn1 -- L foot/LConn1
  R foot/RConn1 -- Rigid Transform8/LConn1 -- Rigid Transform11/RConn1
  Simulink-PS Converter1/RConn1 -- R hip/LConn2
  Rectangular Joint/RConn3 -- PS-Simulink Converter3/LConn1
  L hip/RConn2 -- PS-Simulink Converter/LConn1
  L hip/RConn3 -- PS-Simulink Converter1/LConn1
  R knee/RConn3 -- PS-Simulink Converter11/LConn1
  Brick Solid3/RConn1 -- Rigid Transform5/RConn1
  PS-Simulink Converter7/LConn1 -- Spatial Contact Force1/RConn2
  L knee/LConn1 -- Rigid Transform9/RConn1
  Spatial Contact Force2/RConn1 -- R foot/LConn1
  R hip/RConn3 -- PS-Simulink Converter9/LConn1
  PS-Simulink Converter12/LConn1 -- Spatial Contact Force2/RConn2
  Rigid Transform7/LConn1 -- Rigid Transform10/RConn1
  Rectangular Joint/RConn2 -- PS-Simulink Converter2/LConn1
  Rigid Transform5/LConn1 -- Rigid Transform7/RConn1 -- L foot/RConn1
  R knee/RConn2 -- PS-Simulink Converter10/LConn1
  L knee/RConn2 -- PS-Simulink Converter4/LConn1
  Rigid Transform11/LConn1 -- Rigid Transform4/RConn1
  Rigid Transform10/LConn1 -- L knee/RConn1
  R hip/RConn2 -- PS-Simulink Converter8/LConn1
  R knee/LConn1 -- Rigid Transform12/RConn1
  R knee/LConn2 -- Simulink-PS Converter3/RConn1
  Rigid Transform9/LConn1 -- Rigid Transform1/RConn1
  Rigid Transform4/LConn1 -- R knee/RConn1
  L knee/LConn2 -- Simulink-PS Converter4/RConn1
  Rigid Transform2/LConn1 -- L hip/RConn1 -- Rigid Transform1/LConn1

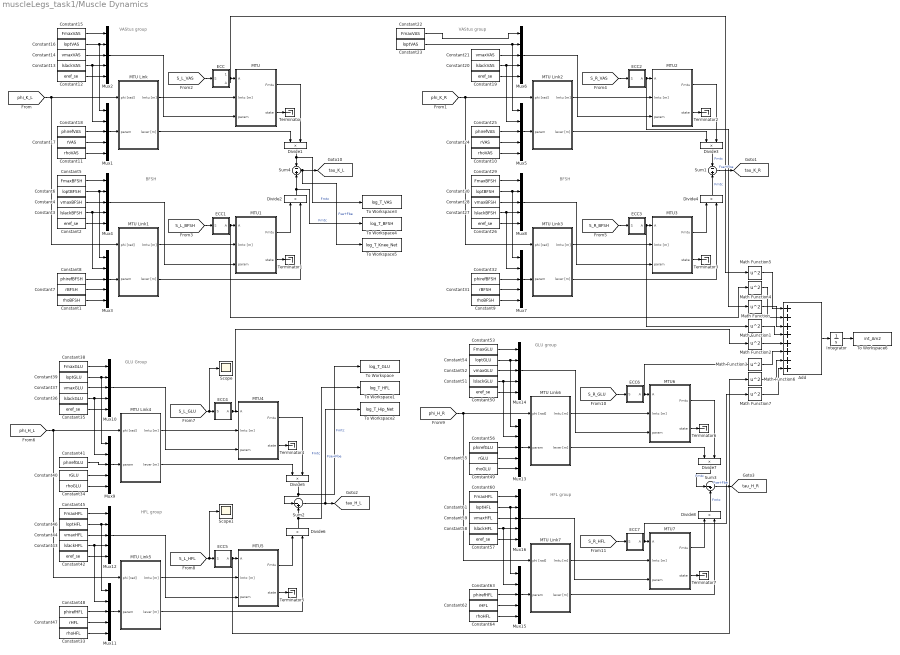
== system muscleLegs_task1/Muscle Dynamics ==
  note: VAStus group
  note: BFSH
  note: VAStus group
  note: BFSH
  note: GLU Group
  note: HFL group
  note: HFL group
  note: GLU group
  Add : Sum  Inputs=++++++++
  Constant1 : Constant  Value=rhoBFSH
  Constant10 : Constant  Value=rhoVAS
  Constant11 : Constant  Value=rhoVAS
  Constant{2,12,19,26,35,42,50,57} (8 alike) : Constant  Value=eref_se
  Constant13 : Constant  Value=lslackVAS
  Constant14 : Constant  Value=vmaxVAS
  Constant15 : Constant  Value=FmaxVAS
  Constant16 : Constant  Value=loptVAS
  Constant17 : Constant  Value=rVAS
  Constant18 : Constant  Value=phirefVAS
  Constant20 : Constant  Value=lslackVAS
  Constant21 : Constant  Value=vmaxVAS
  Constant22 : Constant  Value=FmaxVAS
  Constant23 : Constant  Value=loptVAS
  Constant24 : Constant  Value=rVAS
  Constant25 : Constant  Value=phirefVAS
  Constant27 : Constant  Value=lslackBFSH
  Constant28 : Constant  Value=vmaxBFSH
  Constant29 : Constant  Value=FmaxBFSH
  Constant3 : Constant  Value=lslackBFSH
  Constant30 : Constant  Value=loptBFSH
  Constant31 : Constant  Value=rBFSH
  Constant32 : Constant  Value=phirefBFSH
  Constant33 : Constant  Value=rhoHFL
  Constant34 : Constant  Value=rhoGLU
  Constant36 : Constant  Value=lslackGLU
  Constant37 : Constant  Value=vmaxGLU
  Constant38 : Constant  Value=FmaxGLU
  Constant39 : Constant  Value=loptGLU
  Constant4 : Constant  Value=vmaxBFSH
  Constant40 : Constant  Value=rGLU
  Constant41 : Constant  Value=phirefGLU
  Constant43 : Constant  Value=lslackHFL
  Constant44 : Constant  Value=vmaxHFL
  Constant45 : Constant  Value=FmaxHFL
  Constant46 : Constant  Value=loptHFL
  Constant47 : Constant  Value=rHFL
  Constant48 : Constant  Value=phirefHFL
  Constant49 : Constant  Value=rhoGLU
  Constant5 : Constant  Value=FmaxBFSH
  Constant51 : Constant  Value=lslackGLU
  Constant52 : Constant  Value=vmaxGLU
  Constant53 : Constant  Value=FmaxGLU
  Constant54 : Constant  Value=loptGLU
  Constant55 : Constant  Value=rGLU
  Constant56 : Constant  Value=phirefGLU
  Constant58 : Constant  Value=lslackHFL
  Constant59 : Constant  Value=vmaxHFL
  Constant6 : Constant  Value=loptBFSH
  Constant60 : Constant  Value=FmaxHFL
  Constant61 : Constant  Value=loptHFL
  Constant62 : Constant  Value=rHFL
  Constant63 : Constant  Value=phirefHFL
  Constant64 : Constant  Value=rhoHFL
  Constant7 : Constant  Value=rBFSH
  Constant8 : Constant  Value=phirefBFSH
  Constant9 : Constant  Value=rhoBFSH
  Divide{1..8} (8 alike) : Product
  ECC : Subsystem
  ECC1 : Subsystem
  ECC2 : Subsystem
  ECC3 : Subsystem
  ECC4 : Subsystem
  ECC5 : Subsystem
  ECC6 : Subsystem
  ECC7 : Subsystem
  Integrator : Integrator
  MTU : Subsystem
  MTU Link : Subsystem
  MTU Link1 : Subsystem
  MTU Link2 : Subsystem
  MTU Link3 : Subsystem
  MTU Link4 : Subsystem
  MTU Link5 : Subsystem
  MTU Link6 : Subsystem
  MTU Link7 : Subsystem
  MTU1 : Subsystem
  MTU2 : Subsystem
  MTU3 : Subsystem
  MTU4 : Subsystem
  MTU5 : Subsystem
  MTU6 : Subsystem
  MTU7 : Subsystem
  Math Function{,1..7} (8 alike) : Math  Operator=square
  Mux{1..16} (16 alike) : Mux  Inputs=5
  Scope : Scope
      settings: ActiveDisplayYMinimum=-0.19072734164298966  ActiveDisplayYMaximum=1.1365182783001846
  Scope1 : Scope
      settings: ActiveDisplayYMinimum=-1  ActiveDisplayYMaximum=1  DataLoggingVariableName=ScopeData3
  Sum1 : Sum  Inputs=-+  InputSameDT=on  SaturateOnIntegerOverflow=on  OutDataTypeStr=Inherit: Same as first input
  Sum2 : Sum  Inputs=|-+  InputSameDT=on  SaturateOnIntegerOverflow=on  OutDataTypeStr=Inherit: Same as first input
  Sum3 : Sum  Inputs=|-+  InputSameDT=on  SaturateOnIntegerOverflow=on  OutDataTypeStr=Inherit: Same as first input
  Sum4 : Sum  Inputs=-+  InputSameDT=on  SaturateOnIntegerOverflow=on  OutDataTypeStr=Inherit: Same as first input
  Terminator{,1..7} (8 alike) : Terminator
  To Workspace : ToWorkspace  VariableName=log_T_GLU  SaveFormat=Timeseries  SampleTime=-1
  To Workspace1 : ToWorkspace  VariableName=log_T_HFL  SaveFormat=Timeseries  SampleTime=-1
  To Workspace2 : ToWorkspace  VariableName=log_T_Hip_Net  SaveFormat=Timeseries  SampleTime=-1
  To Workspace3 : ToWorkspace  VariableName=log_T_VAS  SaveFormat=Timeseries  SampleTime=-1
  To Workspace4 : ToWorkspace  VariableName=log_T_BFSH  SaveFormat=Timeseries  SampleTime=-1
  To Workspace5 : ToWorkspace  VariableName=log_T_Knee_Net  SaveFormat=Timeseries  SampleTime=-1
  To Workspace6 : ToWorkspace  VariableName=int_Am2  SaveFormat=Timeseries  SampleTime=-1
  tag scope: tau_H_L=global, tau_H_R=global, tau_K_L=global, tau_K_R=global
  wires:
  Constant11/1 -> Mux1/5
  MTU/2(state) -> Terminator/1
  Constant18/1 -> Mux1/3
  Mux2/1 -> MTU/3(param)
  Constant13/1 -> Mux1/2, Mux2/4
  Constant17/1 -> Mux1/4
  Mux1/1 -> MTU Link/2(param)
  MTU Link/2(lever [m]) -> Divide1/1
  Constant12/1 -> Mux2/5
  MTU/1(Fmtu) -> Divide1/2
  Constant14/1 -> Mux2/3
  Constant16/1 -> Mux1/1, Mux2/2
  MTU Link/1(lmtu [m]) -> MTU/2(lmtc [m])
  Constant15/1 -> Mux2/1
  [S_L_VAS] -> ECC/1(S)
  Divide1/1 -> To Workspace3/1, Sum4/1  "Fmtc"
  Sum4/1 -> To Workspace5/1, [tau_K_L]  "Fse+Fbe"
  [phi_K_L] -> MTU Link/1(phi [rad]), MTU Link1/1(phi [rad])
  Mux3/1 -> MTU Link1/2(param)
  MTU Link1/1(lmtu [m]) -> MTU1/2(lmtc [m])
  [S_L_BFSH] -> ECC1/1(S)
  Constant5/1 -> Mux4/1
  Constant3/1 -> Mux3/2, Mux4/4
  Constant7/1 -> Mux3/4
  Mux4/1 -> MTU1/3(param)
  Constant8/1 -> Mux3/3
  Constant1/1 -> Mux3/5
  MTU1/2(state) -> Terminator1/1
  Constant2/1 -> Mux4/5
  Constant6/1 -> Mux3/1, Mux4/2
  Constant4/1 -> Mux4/3
  MTU1/1(Fmtu) -> Divide2/1
  MTU Link1/2(lever [m]) -> Divide2/2
  Divide2/1 -> To Workspace4/1, Sum4/2  "Fmtc"
  Divide4/1 -> Sum1/2  "Fmtc"
  [S_R_BFSH] -> ECC3/1(S)
  [phi_K_R] -> MTU Link2/1(phi [rad]), MTU Link3/1(phi [rad])
  Mux5/1 -> MTU Link2/2(param)
  MTU Link2/2(lever [m]) -> Divide3/1
  Constant22/1 -> Mux6/1
  Constant20/1 -> Mux5/2, Mux6/4
  Constant24/1 -> Mux5/4
  Constant25/1 -> Mux5/3
  Constant10/1 -> Mux5/5
  Divide3/1 -> Sum1/1  "Fmtc"
  Constant28/1 -> Mux8/3
  Constant9/1 -> Mux7/5
  Constant30/1 -> Mux7/1, Mux8/2
  MTU3/2(state) -> Terminator3/1
  Constant32/1 -> Mux7/3
  MTU2/2(state) -> Terminator2/1
  Mux8/1 -> MTU3/3(param)
  MTU Link3/2(lever [m]) -> Divide4/2
  MTU Link3/1(lmtu [m]) -> MTU3/2(lmtc [m])
  Constant27/1 -> Mux7/2, Mux8/4
  Constant29/1 -> Mux8/1
  Mux7/1 -> MTU Link3/2(param)
  MTU Link2/1(lmtu [m]) -> MTU2/2(lmtc [m])
  MTU2/1(Fmtu) -> Divide3/2
  Constant19/1 -> Mux6/5
  Mux6/1 -> MTU2/3(param)
  MTU3/1(Fmtu) -> Divide4/1
  Constant26/1 -> Mux8/5
  Constant31/1 -> Mux7/4
  Constant23/1 -> Mux5/1, Mux6/2
  Sum1/1 -> [tau_K_R]  "Fse+Fbe"
  Constant21/1 -> Mux6/3
  ECC1/1(A) -> Math Function4/1, MTU1/1(A)
  [S_R_VAS] -> ECC2/1(S)
  ECC2/1(A) -> Math Function/1, MTU2/1(A)
  ECC3/1(A) -> Math Function1/1, MTU3/1(A)
  MTU4/2(state) -> Terminator4/1
  Constant40/1 -> Mux9/4
  Divide5/1 -> To Workspace/1, Sum2/1  "Fmtc"
  Mux10/1 -> MTU4/3(param)
  MTU Link4/1(lmtu [m]) -> MTU4/2(lmtc [m])
  Constant48/1 -> Mux11/3
  MTU4/1(Fmtu) -> Divide5/2
  MTU5/2(state) -> Terminator5/1
  MTU Link5/2(lever [m]) -> Divide6/2
  Constant36/1 -> Mux9/2, Mux10/4
  ECC5/1(A) -> Math Function6/1, MTU5/1(A)
  Constant41/1 -> Mux9/3
  Constant45/1 -> Mux12/1
  Constant44/1 -> Mux12/3
  MTU Link5/1(lmtu [m]) -> MTU5/2(lmtc [m])
  Divide6/1 -> To Workspace1/1, Sum2/2  "Fmtc"
  MTU5/1(Fmtu) -> Divide6/1
  Constant39/1 -> Mux9/1, Mux10/2
  Constant38/1 -> Mux10/1
  Constant34/1 -> Mux9/5
  [phi_H_L] -> MTU Link4/1(phi [rad]), MTU Link5/1(phi [rad])
  Mux12/1 -> MTU5/3(param)
  Constant43/1 -> Mux11/2, Mux12/4
  [S_L_GLU] -> Scope/1, ECC4/1(S)
  Sum2/1 -> To Workspace2/1, [tau_H_L]  "Fse+Fbe"
  Mux11/1 -> MTU Link5/2(param)
  ECC4/1(A) -> Math Function2/1, MTU4/1(A)
  MTU Link4/2(lever [m]) -> Divide5/1
  Constant46/1 -> Mux11/1, Mux12/2
  Constant35/1 -> Mux10/5
  Constant37/1 -> Mux10/3
  Constant42/1 -> Mux12/5
  Mux9/1 -> MTU Link4/2(param)
  Constant33/1 -> Mux11/5
  Constant47/1 -> Mux11/4
  Constant53/1 -> Mux14/1
  Mux13/1 -> MTU Link6/2(param)
  MTU Link6/1(lmtu [m]) -> MTU6/2(lmtc [m])
  Constant60/1 -> Mux16/1
  Mux16/1 -> MTU7/3(param)
  Mux14/1 -> MTU6/3(param)
  Divide8/1 -> Sum3/2  "Fmtc"
  MTU6/2(state) -> Terminator6/1
  Constant64/1 -> Mux15/5
  Constant59/1 -> Mux16/3
  Constant61/1 -> Mux15/1, Mux16/2
  MTU6/1(Fmtu) -> Divide7/2
  ECC6/1(A) -> Math Function3/1, MTU6/1(A)
  [phi_H_R] -> MTU Link6/1(phi [rad]), MTU Link7/1(phi [rad])
  Constant49/1 -> Mux13/5
  Constant55/1 -> Mux13/4
  Mux15/1 -> MTU Link7/2(param)
  Divide7/1 -> Sum3/1  "Fmtc"
  Constant56/1 -> Mux13/3
  Constant62/1 -> Mux15/4
  Constant54/1 -> Mux13/1, Mux14/2
  [S_R_GLU] -> ECC6/1(S)
  Constant63/1 -> Mux15/3
  Constant52/1 -> Mux14/3
  MTU Link6/2(lever [m]) -> Divide7/1
  ECC7/1(A) -> Math Function7/1, MTU7/1(A)
  Constant57/1 -> Mux16/5
  MTU7/2(state) -> Terminator7/1
  MTU Link7/1(lmtu [m]) -> MTU7/2(lmtc [m])
  Constant50/1 -> Mux14/5
  Constant51/1 -> Mux13/2, Mux14/4
  Sum3/1 -> [tau_H_R]  "Fse+Fbe"
  MTU Link7/2(lever [m]) -> Divide8/2
  MTU7/1(Fmtu) -> Divide8/1
  [S_R_HFL] -> ECC7/1(S)
  Constant58/1 -> Mux15/2, Mux16/4
  [S_L_HFL] -> Scope1/1, ECC5/1(S)
  ECC/2(A) -> Math Function5/1, MTU/1(A)
  Math Function5/1 -> Add/1
  Math Function4/1 -> Add/2
  Math Function/1 -> Add/3
  Math Function1/1 -> Add/4
  Math Function2/1 -> Add/5
  Math Function3/1 -> Add/6
  Math Function6/1 -> Add/7
  Math Function7/1 -> Add/8
  Add/1 -> Integrator/1
  Integrator/1 -> To Workspace6/1
